simulink model "flattening_1_test"  (Simulink 9.0)
settings: Solver=ode3  StartTime=0.0  StopTime=10.0  FixedStep=0.200000  RelTol=1e-3  EnableMultiTasking=on
settings Model: SuppressorTable=22 serialization::archive 11 0 6 0 0 0 0 0  Creator=arnaud  LastModifiedBy=hbourbou
settings DataIOCC: LimitDataPoints=on  SignalLoggingSaveFormat=ModelDataLogs
settings OptimizationCC: ExpressionDepthLimit=2147483647
settings DebuggingCC: SolverPrmCheckMsg=warning  FcnCallInpInsideContextMsg=warning  StateNameClashWarn=warning  StrictBusMsg=Warning
settings GRTTargetCC: CombineOutputUpdateFcns=off  GRTInterface=on

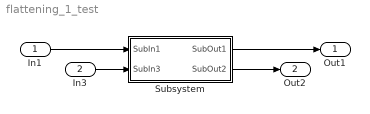
== system flattening_1_test ==
  In1 : Inport
  In3 : Inport  Port=2
  Subsystem : Subsystem
  Out1 : Outport
  Out2 : Outport  Port=2
  wires:
  In1/1 -> Subsystem/1(SubIn1)
  Subsystem/1(SubOut1) -> Out1/1
  In3/1 -> Subsystem/2(SubIn3)
  Subsystem/2(SubOut2) -> Out2/1

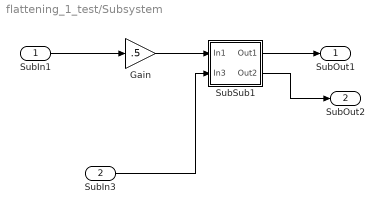
== system flattening_1_test/Subsystem ==
  SubIn1 : Inport
  SubIn3 : Inport  Port=2
  Gain : Gain  Gain=.5
  SubSub1 : Subsystem
  SubOut1 : Outport
  SubOut2 : Outport  Port=2
  wires:
  Gain/1 -> SubSub1/1(In1)
  SubSub1/1(Out1) -> SubOut1/1
  SubIn1/1 -> Gain/1
  SubIn3/1 -> SubSub1/2(In3)
  SubSub1/2(Out2) -> SubOut2/1

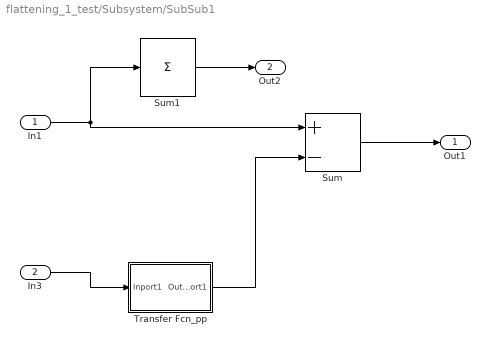
== system flattening_1_test/Subsystem/SubSub1 ==
  In1 : Inport
  In3 : Inport  Port=2
  Sum : Sum  Inputs=+-
  Sum1 : Sum  Inputs=+
  Transfer Fcn_pp : Subsystem
  Out1 : Outport
  Out2 : Outport  Port=2
  wires:
  In3/1 -> Transfer Fcn_pp/1(Inport1)
  Sum/1 -> Out1/1
  In1/1 -> Sum1/1, Sum/1
  Transfer Fcn_pp/1(Outport1) -> Sum/2
  Sum1/1 -> Out2/1

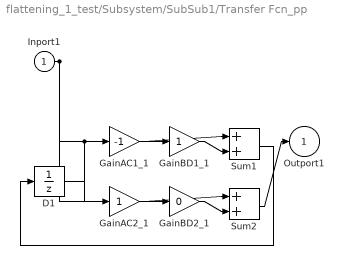
== system flattening_1_test/Subsystem/SubSub1/Transfer Fcn_pp ==
  Inport1 : Inport
  D1 : UnitDelay  SampleTime=-1
  GainAC1_1 : Gain  Gain=-1  SaturateOnIntegerOverflow=on  OutDataTypeStr=Inherit: Same as input  ParamDataTypeStr=Inherit: Same as input
  GainAC2_1 : Gain  SaturateOnIntegerOverflow=on  OutDataTypeStr=Inherit: Same as input  ParamDataTypeStr=Inherit: Same as input
  GainBD1_1 : Gain  SaturateOnIntegerOverflow=on  OutDataTypeStr=Inherit: Same as input  ParamDataTypeStr=Inherit: Same as input
  GainBD2_1 : Gain  Gain=0  SaturateOnIntegerOverflow=on  OutDataTypeStr=Inherit: Same as input  ParamDataTypeStr=Inherit: Same as input
  Sum1 : Sum  SaturateOnIntegerOverflow=on  InputSameDT=on  OutDataTypeStr=Inherit: Same as first input
  Sum2 : Sum  SaturateOnIntegerOverflow=on  InputSameDT=on  OutDataTypeStr=Inherit: Same as first input
  Outport1 : Outport
  wires:
  D1/1 -> GainAC1_1/1, GainAC2_1/1
  GainAC1_1/1 -> Sum1/1
  GainAC2_1/1 -> Sum2/1
  Inport1/1 -> GainBD1_1/1, GainBD2_1/1
  GainBD1_1/1 -> Sum1/2
  GainBD2_1/1 -> Sum2/2
  Sum1/1 -> D1/1
  Sum2/1 -> Outport1/1
